simulink model "lab2_MC"  (Simulink 8.9)
settings: Solver=ode3  StartTime=0.0  StopTime=1000  FixedStep=1  RelTol=1e-3  EnableMultiTasking=on
undefined symbols (not defined in the file or in its folder): DiscIntNeverNeededParam
libraries: simulink x1
settings Model: Creator=IEUser  LastModifiedBy=igorkislyuk
settings OptimizationCC: BooleanDataType=off  ExpressionDepthLimit=2147483647
settings DebuggingCC: SolverPrmCheckMsg=warning
settings GRTTargetCC: GeneratePreprocessorConditionals=Use local settings

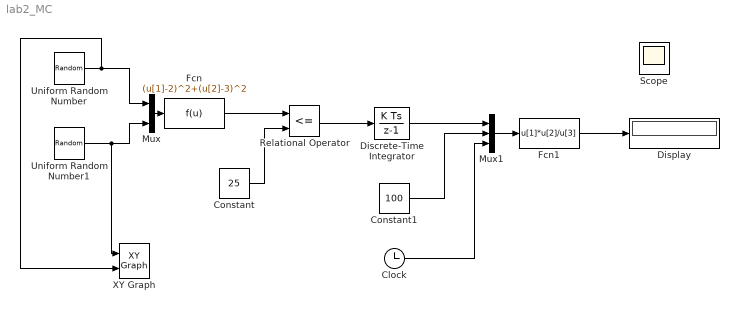
== system lab2_MC ==
  Clock : Clock
  Constant : Constant  Value=25
  Constant1 : Constant  Value=100
  Discrete-Time Integrator : DiscreteIntegrator  OutDataTypeStr=double  ICPrevOutput=DiscIntNeverNeededParam  ICPrevScaledInput=DiscIntNeverNeededParam
  Display : Display
  Fcn : Fcn  Expr=(u[1]-2)^2+(u[2]-3)^2
  Fcn1 : Fcn  Expr=u[1]*u[2]/u[3]
  Mux : Mux  Inputs=2
  Mux1 : Mux  Inputs=3
  Relational Operator : RelationalOperator  Operator=<=  OutDataTypeStr=boolean  RndMeth=Nearest
  Scope : Scope
  Uniform Random Number : UniformRandomNumber  Minimum=-3  Maximum=7  SampleTime=0
  Uniform Random Number1 : UniformRandomNumber  Minimum=-2  Maximum=8  Seed=11  SampleTime=0
  XY Graph : simulink/Sinks/XY Graph  xmin=-2  xmax=8  ymin=-2  ymax=8  st=0
  wires:
  Uniform Random Number/1 -> XY Graph/2, Mux/1
  Uniform Random Number1/1 -> XY Graph/1, Mux/2
  Mux/1 -> Fcn/1
  Constant/1 -> Relational Operator/2
  Fcn/1 -> Relational Operator/1
  Relational Operator/1 -> Discrete-Time Integrator/1
  Discrete-Time Integrator/1 -> Mux1/1
  Constant1/1 -> Mux1/2
  Clock/1 -> Mux1/3
  Mux1/1 -> Fcn1/1
  Fcn1/1 -> Display/1
